simulink library "dgcmgFourParallelArray_sl"  (R2024b)
settings: Solver=VariableStepAuto  StartTime=0.0  StopTime=10.0  RelTol=1e-3
undefined symbols (not defined in the file): gimbalAngRate0, gimbalAngRates0, rotorAngRate, rotorInertia
libraries: simulink x1
settings Model: Creator=gilbu
settings RTWCC: GPUComputeCapability=3.5

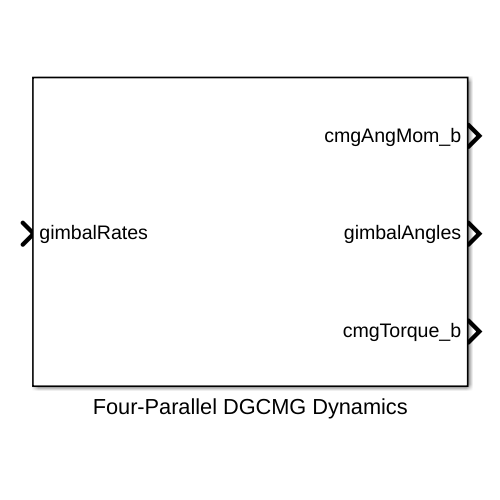
[thumbnail: Simulink's stored preview of the top-level diagram]
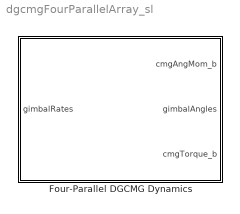
== system dgcmgFourParallelArray_sl ==
  Four-Parallel DGCMG Dynamics : Subsystem  mask{rotorInertia=rotorInertia, rotorAngRate=rotorAngRate, Parameter3=gimbalAngRates0}
      mask prompts: rotorInertia "CMG Rotor Moment of Inertia <1> [kg*m2]"; rotorAngRate "CMG Rotor Angular Rate <1> [rad/s]"; Parameter3 "Initial gimbal angles <8> [rad/s]"
      mask DialogControl DescTextVar Prompt: Hardware Model for a four double gimbal CMG array mounted in a parallel configuration. The input gimbalRates should be an 8 by 1 vector with formatted as [a1,b1,a2,b2,...].

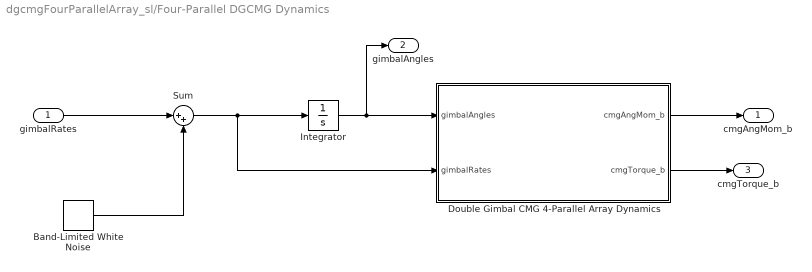
== system dgcmgFourParallelArray_sl/Four-Parallel DGCMG Dynamics ==
  gimbalRates : Inport
  Band-Limited White Noise : simulink/Sources/Band-Limited White Noise  Cov=[1e-8]  Ts=0.1  seed=[23341]
  Double Gimbal CMG 4-Parallel Array Dynamics : MATLAB Function  TreatAsAtomicUnit=on
  Integrator : Integrator  InitialCondition=gimbalAngRate0
  Sum : Sum  Inputs=|++
  cmgAngMom_b : Outport
  gimbalAngles : Outport  Port=2  PortDimensions=8
  cmgTorque_b : Outport  Port=3
  wires:
  Integrator/1 -> gimbalAngles/1, Double Gimbal CMG 4-Parallel Array Dynamics/1(gimbalAngles)
  Double Gimbal CMG 4-Parallel Array Dynamics/1(cmgAngMom_b) -> cmgAngMom_b/1
  Double Gimbal CMG 4-Parallel Array Dynamics/2(cmgTorque_b) -> cmgTorque_b/1
  Band-Limited White Noise/1 -> Sum/2
  gimbalRates/1 -> Sum/1
  Sum/1 -> Double Gimbal CMG 4-Parallel Array Dynamics/2(gimbalRates), Integrator/1

== matlab function dgcmgFourParallelArray_sl/Four-Parallel DGCMG Dynamics/Double Gimbal CMG 4-Parallel Array Dynamics ==
  data: gimbalAngles input size=8; gimbalRates input size=8; cmgAngMom_b output size=3; rotorInertia parameter size=1; rotorAngRate parameter size=1; cmgTorque_b output size=3
%dgcmgDynamics  Dynamics for 4 paralle mounted Doule Gimbal CMG
% Author: Antonio Gil Buitragos
function [cmgAngMom_b,cmgTorque_b]  = dcmgDynamics( ...
   gimbalAngles,gimbalRates,... %Inputs
   rotorInertia, rotorAngRate)          ... %Parameters
%------------------------------------------------------------------------------
% CMG Dynamics from Space Vehicle Dynamics-Bong Wie

%-------------------------------------------------------------------------------
% Initialize Variables

% Rotor Angular Momentum
rotorAngMom = rotorInertia*rotorAngRate;

% Trig Functions
sa1 = sin(gimbalAngles(1));
ca1 = cos(gimbalAngles(1));
cb1 = cos(gimbalAngles(2));
sb1 = sin(gimbalAngles(2));

sa2 = sin(gimbalAngles(3));
ca2 = cos(gimbalAngles(3));
cb2 = cos(gimbalAngles(4));
sb2 = sin(gimbalAngles(4));

sa3 = sin(gimbalAngles(5));
ca3 = cos(gimbalAngles(5));
cb3 = cos(gimbalAngles(6));
sb3 = sin(gimbalAngles(6));

sa4 = sin(gimbalAngles(7));
ca4 = cos(gimbalAngles(7));
cb4 = cos(gimbalAngles(8));
sb4 = sin(gimbalAngles(8));

% Gimbal Direction Matrix
C = [sa1 sa2 sa3 sa4;
     cb1*ca1 cb1*ca2 cb3*ca3 cb4*ca4;
     sb1*ca1 sb2*ca2 sb3*ca3 sb4*ca4];


%-------------------------------------------------------------------------------
% CMG Dynamics

% Angular Momentum
cmgAngMom_b = rotorAngMom*C(:,1)+rotorAngMom*C(:,2)+rotorAngMom*C(:,3)+rotorAngMom*C(:,4);

% DGCMG_i Torque. GimbalRates: Even index are alpha_i. Odd index are beta_i.
hDotG1 = [ca1*gimbalRates(1) -sa1*cb1*gimbalRates(1)-ca1*sb1*gimbalRates(2) -sa1*sb1*gimbalRates(1)+ca1*cb1*gimbalRates(2)]';
hDotG2 = [ca2*gimbalRates(3) -sa2*cb2*gimbalRates(3)-ca2*sb2*gimbalRates(4) -sa2*sb2*gimbalRates(3)+ca2*cb2*gimbalRates(4)]';
hDotG3 = [ca3*gimbalRates(5) -sa3*cb3*gimbalRates(5)-ca3*sb3*gimbalRates(6) -sa3*sb3*gimbalRates(5)+ca3*cb3*gimbalRates(6)]';
hDotG4 = [ca4*gimbalRates(7) -sa4*cb4*gimbalRates(7)-ca4*sb4*gimbalRates(8) -sa4*sb4*gimbalRates(7)+ca4*cb4*gimbalRates(8)]';


% Total CMG Array Output Torque.
cmgTorque_b = rotorAngMom.*(hDotG1+hDotG2+hDotG3+hDotG4);



%-------------------------------------------------------------------------------
end
